simulink model "example_controller"  (R2018b)
settings: Solver=FixedStepDiscrete  StartTime=0.0  StopTime=inf  FixedStep=sample_time  RelTol=1e-3
InitFcn:
  | addpath('../common/')
  | simulation_params
  | mechanical_params
values from neighbouring files (symbols this model uses):
  sample_time = 1/sample_freq    (= 0.001)    [simulation_params.m]
settings Model: Creator=wmartin  LastModifiedBy=ixido
settings DataIOCC: SaveFormat=StructureWithTime  SaveOutput=off  SignalLogging=off  DSMLogging=off  SaveTime=off
settings OptimizationCC: BlockReduction=off  DefaultParameterBehavior=Inlined  UseFloatMulNetSlope=on  InlineInvariantSignals=on  OptimizeBlockIOStorage=off  BufferReuse=off  GlobalBufferReuse=off  ExpressionFolding=off  LocalBlockOutputs=off  LifeSpan=0.5  SimCompilerOptimization=on  OptimizeDataStoreBuffers=off  BusAssignmentInplaceUpdate=off
settings DebuggingCC: UnderspecifiedInitializationDetection=Classic  MergeDetectMultiDrivingBlocksExec=none  LibraryContextMissingDiagnostic=none
settings HardwareCC: ProdBitPerPointer=32  ProdBitPerSizeT=32  ProdBitPerPtrDiffT=32  ProdLargestAtomicFloat=None  ProdWordSize=32  ProdLongLongMode=on  ProdHWDeviceType=Generic->32-bit x86 compatible
settings ModelReferenceCC: ModelReferenceNumInstancesAllowed=Single  ModelReferenceMinAlgLoopOccurrences=on  PropagateSignalLabelsOutOfModel=off
settings SFSimCC: SimUseLocalCustomCode=off
settings RTWCC: SystemTargetFile=slrt.tlc  TLCOptions=-axPCModelStackSizeKB=1024  TemplateMakefile=slrt_default_tmf  Description=Simulink Real-Time  RTWUseLocalCustomCode=off  CodeExecutionProfiling=on  RTWCompilerOptimization=on
settings CodeAppCC: MaxIdLength=127  StateflowObjectComments=on
settings TargetCC: CodeReplacementLibrary=XPC_BLAS  ParMdlRefBuildCompliant=on  ConcurrentExecutionCompliant=on  GeneratePreprocessorConditionals=Use local settings  MatFileLogging=on  PreserveStateflowLocalDataDimensions=off  MATLABClassNameForMDSCustomization=xpcAperiodicCustomization

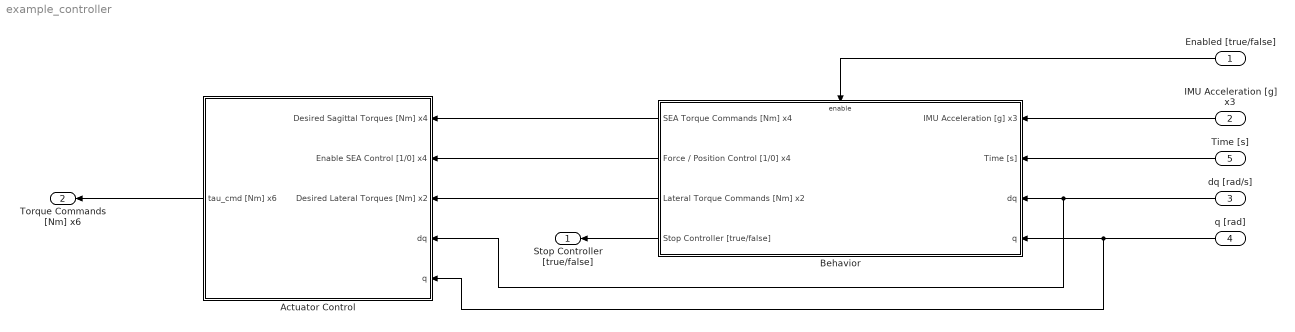
== system example_controller ==
  Enabled [true/false] : Inport  OutDataTypeStr=boolean  PortDimensions=1  SampleTime=sample_time  Interpolate=off
  IMU Acceleration [g] x3 : Inport  Port=2  OutDataTypeStr=double  PortDimensions=3  SampleTime=[0.001,0]  Interpolate=off
  dq [rad/s] : Inport  Port=3  OutDataTypeStr=double  PortDimensions=13  SampleTime=[0.001,0]  Interpolate=off
  q [rad] : Inport  Port=4  OutDataTypeStr=double  PortDimensions=13  SampleTime=[0.001,0]  Interpolate=off
  Time [s] : Inport  Port=5  OutDataTypeStr=double  PortDimensions=1  SampleTime=sample_time  Interpolate=off
  Actuator Control : Subsystem
  Behavior : Subsystem
  Stop Controller [true/false] : Outport  OutDataTypeStr=boolean  PortDimensions=1  SampleTime=[0.001,0]  OutputWhenDisabled=reset  InitialOutput=[0 0 0 0 0 0]
  Torque Commands [Nm] x6 : Outport  Port=2  OutDataTypeStr=double  PortDimensions=6  SampleTime=[0.001,0]  OutputWhenDisabled=reset  InitialOutput=[0 0 0 0 0 0]
  wires:
  IMU Acceleration [g] x3/1 -> Behavior/1(IMU Acceleration [g] x3)
  dq [rad/s]/1 -> Behavior/3(dq), Actuator Control/4(dq)
  q [rad]/1 -> Behavior/4(q), Actuator Control/5(q)
  Time [s]/1 -> Behavior/2(Time [s])
  Enabled [true/false]/1 -> Behavior/Enable
  Behavior/4(Stop Controller [true/false]) -> Stop Controller [true/false]/1
  Behavior/2(Force / Position Control [1/0] x4) -> Actuator Control/2(Enable SEA Control [1/0] x4)
  Actuator Control/1(tau_cmd [Nm] x6) -> Torque Commands [Nm] x6/1
  Behavior/1(SEA Torque Commands [Nm] x4) -> Actuator Control/1(Desired Sagittal Torques [Nm] x4)
  Behavior/3(Lateral Torque Commands [Nm] x2) -> Actuator Control/3(Desired Lateral Torques [Nm] x2)

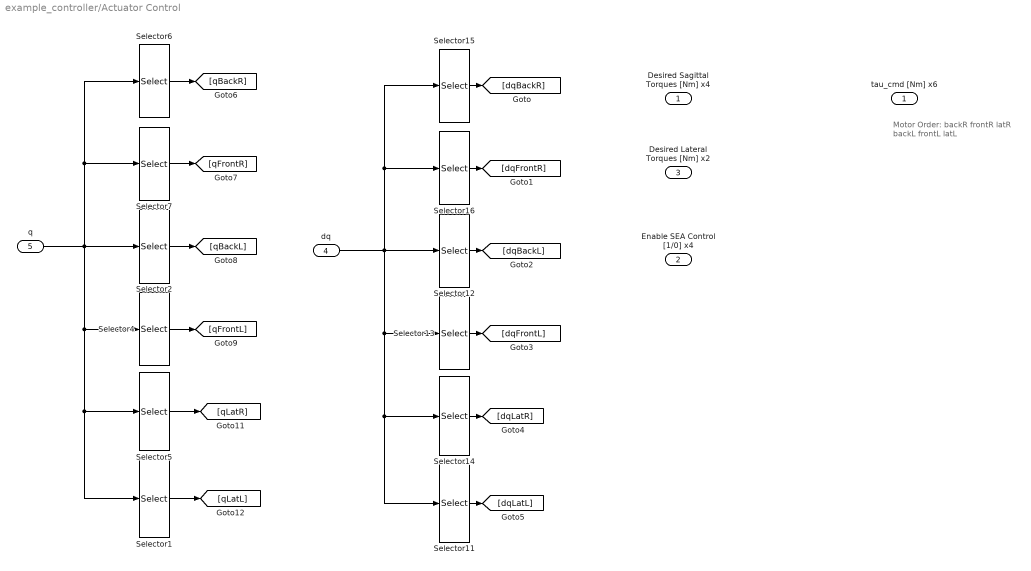
== system example_controller/Actuator Control ==
  note: Motor Order:
      |
      | backR
      | frontR
      | latR
      | backL
      | frontL
      | latL
  Desired Sagittal Torques [Nm] x4 : Inport  OutDataTypeStr=double  PortDimensions=4  SampleTime=sample_time
  Enable SEA Control [1/0] x4 : Inport  Port=2  OutDataTypeStr=boolean  PortDimensions=4  SampleTime=sample_time
  Desired Lateral Torques [Nm] x2 : Inport  Port=3  OutDataTypeStr=double  PortDimensions=2  SampleTime=sample_time
  dq : Inport  Port=4  OutDataTypeStr=double  PortDimensions=13  SampleTime=sample_time
  q : Inport  Port=5  OutDataTypeStr=double  PortDimensions=13  SampleTime=sample_time
  Selector1 : Selector  InputPortWidth=13  IndexOptions=Index vector (dialog)  Indices=[10]  OutputSizes=1
  Selector11 : Selector  InputPortWidth=13  IndexOptions=Index vector (dialog)  Indices=[10]  OutputSizes=1
  Selector12 : Selector  InputPortWidth=13  IndexOptions=Index vector (dialog)  Indices=[5 6]  OutputSizes=1
  Selector13 : Selector  InputPortWidth=13  IndexOptions=Index vector (dialog)  Indices=[7 8]  OutputSizes=1
  Selector14 : Selector  InputPortWidth=13  IndexOptions=Index vector (dialog)  Indices=[9]  OutputSizes=1
  Selector15 : Selector  InputPortWidth=13  IndexOptions=Index vector (dialog)  Indices=[1 2]  OutputSizes=1
  Selector16 : Selector  InputPortWidth=13  IndexOptions=Index vector (dialog)  Indices=[3 4]  OutputSizes=1
  Selector2 : Selector  InputPortWidth=13  IndexOptions=Index vector (dialog)  Indices=[5 6]  OutputSizes=1
  Selector4 : Selector  InputPortWidth=13  IndexOptions=Index vector (dialog)  Indices=[7 8]  OutputSizes=1
  Selector5 : Selector  InputPortWidth=13  IndexOptions=Index vector (dialog)  Indices=[9]  OutputSizes=1
  Selector6 : Selector  InputPortWidth=13  IndexOptions=Index vector (dialog)  Indices=[1 2]  OutputSizes=1
  Selector7 : Selector  InputPortWidth=13  IndexOptions=Index vector (dialog)  Indices=[3 4]  OutputSizes=1
  tau_cmd [Nm] x6 : Outport  OutDataTypeStr=double  PortDimensions=6  InitialOutput=[0 0 0 0 0 0]
  wires:
  Selector15/1 -> [dqBackR]
  Selector13/1 -> [dqFrontL]
  Selector1/1 -> [qLatL]
  Selector12/1 -> [dqBackL]
  Selector2/1 -> [qBackL]
  Selector4/1 -> [qFrontL]
  Selector5/1 -> [qLatR]
  Selector6/1 -> [qBackR]
  dq/1 -> Selector12/1, Selector16/1, Selector15/1, Selector13/1, Selector14/1, Selector11/1
  Selector11/1 -> [dqLatL]
  q/1 -> Selector1/1, Selector5/1, Selector4/1, Selector6/1, Selector7/1, Selector2/1
  Selector7/1 -> [qFrontR]
  Selector16/1 -> [dqFrontR]
  Selector14/1 -> [dqLatR]

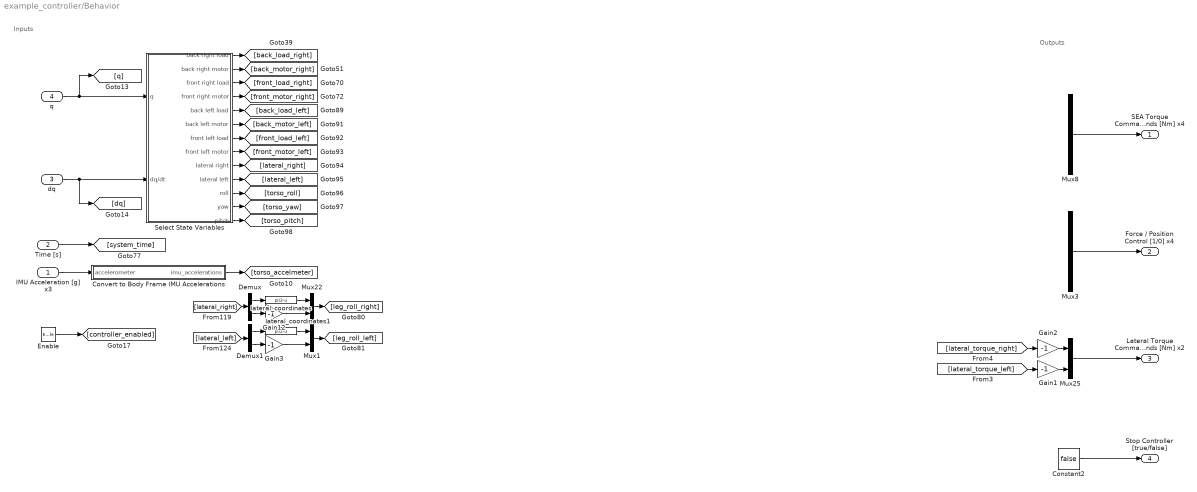
== system example_controller/Behavior ==
  note: Outputs
  note: Inputs
  IMU Acceleration [g] x3 : Inport  OutDataTypeStr=double  PortDimensions=3  SampleTime=[0.001,0]
  Time [s] : Inport  Port=2  OutDataTypeStr=double  PortDimensions=1  SampleTime=[0.001,0]
  dq : Inport  Port=3  OutDataTypeStr=double  PortDimensions=13  SampleTime=[0.001,0]
  q : Inport  Port=4  OutDataTypeStr=double  PortDimensions=13  SampleTime=[0.001,0]
  Enable : EnablePort  PropagateVarSize=During execution  ShowOutputPort=on
  Constant2 : Constant  Value=false
  Convert to Body Frame IMU Accelerations : MATLAB Function  TreatAsAtomicUnit=on
  Demux : Demux  Outputs=2
  Demux1 : Demux  Outputs=2
  Gain{1..3,12} (4 alike) : Gain  Gain=-1
  Mux1 : Mux  Inputs=2
  Mux22 : Mux  Inputs=2
  Mux25 : Mux  Inputs=2
  Mux3 : Mux
  Mux8 : Mux
  Select State Variables : Subsystem
  lateral_coordinates : Fcn  Expr=pi/2-u
  lateral_coordinates1 : Fcn  Expr=pi/2-u
  SEA Torque Commands [Nm] x4 : Outport  OutDataTypeStr=double  PortDimensions=4  SampleTime=[0.001,0]  OutputWhenDisabled=reset  InitialOutput=[0 0 0 0]
  Force / Position Control [1/0] x4 : Outport  Port=2  OutDataTypeStr=boolean  PortDimensions=4  SampleTime=[0.001,0]  OutputWhenDisabled=reset  InitialOutput=[0 0 0 0]
  Lateral Torque Commands [Nm] x2 : Outport  Port=3  OutDataTypeStr=double  PortDimensions=2  SampleTime=[0.001,0]  OutputWhenDisabled=reset  InitialOutput=[0 0]
  Stop Controller [true/false] : Outport  Port=4  OutDataTypeStr=boolean  PortDimensions=1  SampleTime=[0.001,0]  OutputWhenDisabled=reset  InitialOutput=0
  wires:
  Time [s]/1 -> [system_time]
  Demux/2 -> Gain12/1
  lateral_coordinates/1 -> Mux22/1
  Gain12/1 -> Mux22/2
  Mux22/1 -> [leg_roll_right]
  Demux/1 -> lateral_coordinates/1
  [lateral_torque_right] -> Gain2/1
  q/1 -> [q], Select State Variables/1(q)
  [lateral_torque_left] -> Gain1/1
  Mux8/1 -> SEA Torque Commands [Nm] x4/1
  Mux3/1 -> Force / Position Control [1/0] x4/1
  Gain2/1 -> Mux25/1
  Mux25/1 -> Lateral Torque Commands [Nm] x2/1
  Gain1/1 -> Mux25/2
  Constant2/1 -> Stop Controller [true/false]/1
  dq/1 -> [dq], Select State Variables/2(dq/dt)
  Select State Variables/1(back right load) -> [back_load_right]
  Select State Variables/2(back right motor) -> [back_motor_right]
  Select State Variables/3(front right load) -> [front_load_right]
  Select State Variables/4(front right motor) -> [front_motor_right]
  Select State Variables/5(back left load) -> [back_load_left]
  Select State Variables/6(back left motor) -> [back_motor_left]
  Select State Variables/7(front left load) -> [front_load_left]
  Select State Variables/8(front left motor) -> [front_motor_left]
  Select State Variables/13(pitch) -> [torso_pitch]
  Select State Variables/12(yaw) -> [torso_yaw]
  Select State Variables/11(roll) -> [torso_roll]
  Select State Variables/10(lateral left) -> [lateral_left]
  Select State Variables/9(lateral right) -> [lateral_right]
  [lateral_right] -> Demux/1
  [lateral_left] -> Demux1/1
  Demux1/1 -> lateral_coordinates1/1
  Mux1/1 -> [leg_roll_left]
  Gain3/1 -> Mux1/2
  lateral_coordinates1/1 -> Mux1/1
  Demux1/2 -> Gain3/1
  Enable/1 -> [controller_enabled]
  Convert to Body Frame IMU Accelerations/1(imu_accelerations) -> [torso_accelmeter]
  IMU Acceleration [g] x3/1 -> Convert to Body Frame IMU Accelerations/1(accelerometer)

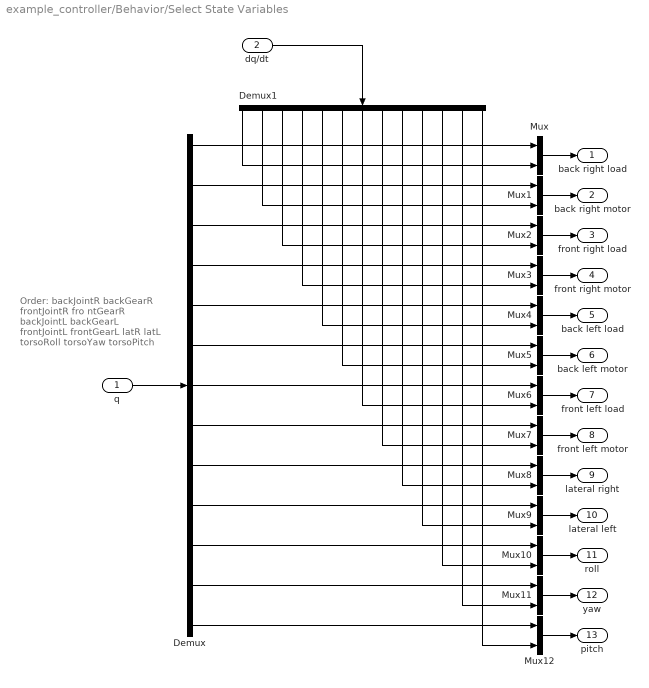
== system example_controller/Behavior/Select State Variables ==
  note: Order:
      |
      | backJointR
      | backGearR
      | frontJointR
      | fro ntGearR
      |
      | backJointL
      | backGearL
      | frontJointL
      | frontGearL
      |
      | latR
      | latL
      |
      | torsoRoll
      | torsoYaw
      | torsoPitch
  q : Inport
  dq/dt : Inport  Port=2
  Demux : Demux  Outputs=13
  Demux1 : Demux  Outputs=13
  Mux{,1..12} (13 alike) : Mux  Inputs=2
  back right load : Outport
  back right motor : Outport  Port=2
  front right load : Outport  Port=3
  front right motor : Outport  Port=4
  back left load : Outport  Port=5
  back left motor : Outport  Port=6
  front left load : Outport  Port=7
  front left motor : Outport  Port=8
  lateral right : Outport  Port=9
  lateral left : Outport  Port=10
  roll : Outport  Port=11
  yaw : Outport  Port=12
  pitch : Outport  Port=13
  wires:
  q/1 -> Demux/1
  dq/dt/1 -> Demux1/1
  Mux/1 -> back right load/1
  Mux1/1 -> back right motor/1
  Mux4/1 -> back left load/1
  Mux5/1 -> back left motor/1
  Mux8/1 -> lateral right/1
  Mux9/1 -> lateral left/1
  Mux12/1 -> pitch/1
  Mux2/1 -> front right load/1
  Mux3/1 -> front right motor/1
  Mux6/1 -> front left load/1
  Mux7/1 -> front left motor/1
  Mux10/1 -> roll/1
  Mux11/1 -> yaw/1
  Demux/1 -> Mux/1
  Demux1/1 -> Mux/2
  Demux/2 -> Mux1/1
  Demux/3 -> Mux2/1
  Demux/4 -> Mux3/1
  Demux/5 -> Mux4/1
  Demux/6 -> Mux5/1
  Demux/7 -> Mux6/1
  Demux/8 -> Mux7/1
  Demux/9 -> Mux8/1
  Demux/10 -> Mux9/1
  Demux/11 -> Mux10/1
  Demux/12 -> Mux11/1
  Demux/13 -> Mux12/1
  Demux1/2 -> Mux1/2
  Demux1/3 -> Mux2/2
  Demux1/4 -> Mux3/2
  Demux1/5 -> Mux4/2
  Demux1/6 -> Mux5/2
  Demux1/7 -> Mux6/2
  Demux1/8 -> Mux7/2
  Demux1/9 -> Mux8/2
  Demux1/10 -> Mux9/2
  Demux1/11 -> Mux10/2
  Demux1/12 -> Mux11/2
  Demux1/13 -> Mux12/2

== matlab function example_controller/Behavior/Convert to Body Frame IMU Accelerations ==
  data: accelerometer input; imu_accelerations output
function imu_accelerations = imu_to_body_frame(accelerometer)
    g = 9.803;
    z_up_rotation = [1, 0, 0; 0, 0, 1; 0, -1, 0];
    align_xy_rotation = [sqrt(2)/2, -sqrt(2)/2, 0; sqrt(2)/2, sqrt(2)/2, 0; 0, 0, 1];
    imu_accelerations = g*z_up_rotation*align_xy_rotation*accelerometer;
end
